simulink model "Receive_Ethernet2024a_UDP"  (R2024b)
settings: Solver=FixedStepAuto  StartTime=0.0  StopTime=inf  FixedStep=0.01  RelTol=1e-3
undefined symbols (not defined in the file): f, gray
libraries: instrumentlib x2, etargetslib x1
settings Model: Creator=hyeon-yongjeong  LastModifiedBy=hyeon-yongjeong

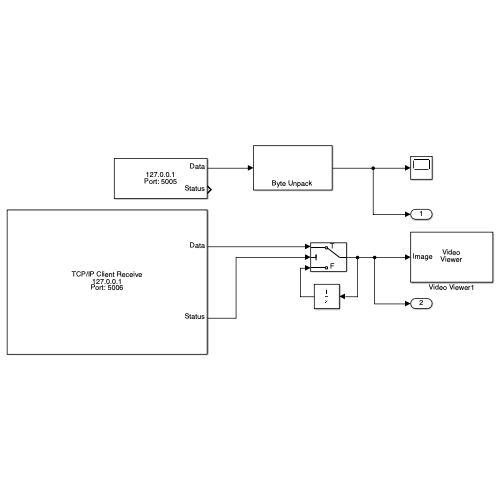
[thumbnail: Simulink's stored preview of the top-level diagram]
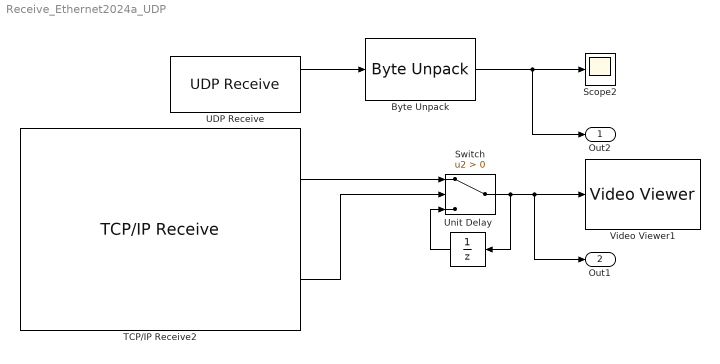
== system Receive_Ethernet2024a_UDP ==
  Byte Unpack : etargetslib/Byte Unpack  dimensions={[9 1]}  datatypes={'double'}  byteAlign=8
      settings: LibrarySourceBlock=embeddedtargetslib/Host Communication/Byte Unpack
  Scope2 : Scope
  Switch : Switch  Criteria=u2 > Threshold  SaturateOnIntegerOverflow=off  InputSameDT=off
  TCP/IP Receive2 : instrumentlib/TCP//IP Receive  Host=127.0.0.1  Port=5006  DataSize=[240 320]  DataType=uint8  ASCIIFormatting=%f  Terminator=LF  CustomTerminator=10  ByteOrder=little-endian  EnableBlockingMode=off  Timeout=10  SampleTime=0.01  SimulateUsing=Interpreted execution
  UDP Receive : instrumentlib/UDP Receive  LocalAddress=127.0.0.1  LocalPort=5005  EnablePortSharing=off  Host=0.0.0.0  Port=5005  GetLatestData=off  DataSize=[8*9 1 ]  DataType=uint8  ASCIIFormatting=%f,  Terminator=LF  CustomTerminator=10  ByteOrder=big-endian  EnableBlockingMode=off  Timeout=10  SampleTime=0.01  SimulateUsing=Interpreted execution
  Unit Delay : UnitDelay  SampleTime=-1  HasFrameUpgradeWarning=on
  Video Viewer1 : VideoViewer  colormapValue=gray(256)  FigPos=[134 753 636 450]
  Out2 : Outport
  Out1 : Outport  Port=2
  wires:
  Byte Unpack/1 -> Scope2/1, Out2/1
  UDP Receive/1 -> Byte Unpack/1
  TCP/IP Receive2/2 -> Switch/2
  Switch/1 -> Unit Delay/1, Out1/1, Video Viewer1/1
  Unit Delay/1 -> Switch/3
  TCP/IP Receive2/1 -> Switch/1
